simulink model "papersimulation"  (R2023b)
settings: Solver=VariableStepAuto  StartTime=0.0  StopTime=50  RelTol=1e-3
InitFcn:
  | clc;clear;close all
  | Aa = [
  |     -0.026373    0.12687    -12.926     -32.169;
  |     -0.25009    -0.80174    220.55      -0.16307;
  |     0.000171    -0.00754    -0.5510     -0.000334;
  |     0           0           1           0
  | ];
  | 
  | ba = [
  |     0.010887;
  |     -0.18577;
  |     -0.022966;
  |     0
  | ];
  | 
  | ca = [
  |     0    0    0    1
  | ];
  | Am=Aa;
  | bm=ba;
  | cm=ca;
  | K1m = [0.003614, -0.306976, 262.056954, 999.941914]';
  | 
  | theta1 = [7.654562; 6.881398; -1.386117];       % 3x1 vector
  | theta2 = [-4434.189351; -5958.822119; -2550.603134]; % 3x1 vector
  | theta20 = 595.409427;                            % Scalar
  | 
  | theta31 = [-7.654459; -6.860858; 1.385877];     % 3x1 vector
  | theta32 = [4434.169641; 5958.808248; 2550.58291]; % 3x1 vector
  | theta33 = -595.40843;                            % Scalar
  | theta34 = 0.998522;
  | theta= [
  |     theta1;
  |     theta2;
  |     theta20;
  |     theta31;
  |     theta32;
  |     theta33;
  |     theta34
  | ];
  | %initial condition
  | theta0=1.1*theta;
  | kp =-0.023;
  | rho0=1.1*kp;
  | %other constant parameters
  | gamma = 5;
  | alpha = 5;
  | Gamma = alpha*eye(length(theta0));
  | sgnkp = -1;
StopFcn:
  | plot(out.tout,out.y,LineWidth=1.5)
  | hold on
  | plot(out.tout,out.ym,LineWidth=1.5)
  | legend(["$y$","$y_m$"],FontSize=18,Interpreter="latex")
  | xlabel("time",FontSize=18,Interpreter="latex")
  | ylim([-0.5 0.5])
  | grid on
  | 
  | figure
  | plot(out.tout,out.u,LineWidth=1.5)
  | legend("Control signal",FontSize=18,Interpreter="latex")
  | xlabel("time",FontSize=18,Interpreter="latex")
  | grid on
  | 
  | figure
  | plot(out.tout,out.e,LineWidth=1.5)
  | legend("Error",FontSize=18,Interpreter="latex")
  | xlabel("time",FontSize=18,Interpreter="latex")
  | ylim([-0.2 0.6])
  | grid on
settings Model: Creator=IHC  LastModifiedBy=IHC

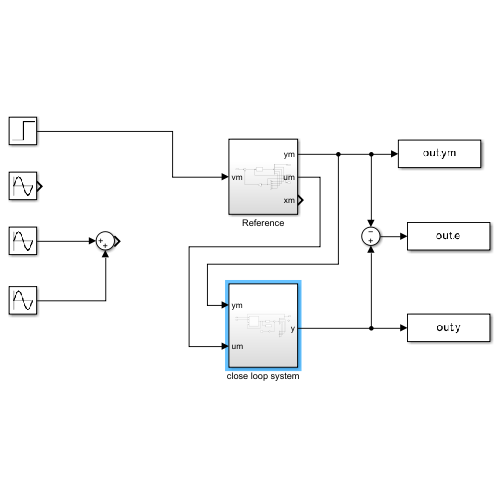
[thumbnail: Simulink's stored preview of the top-level diagram]
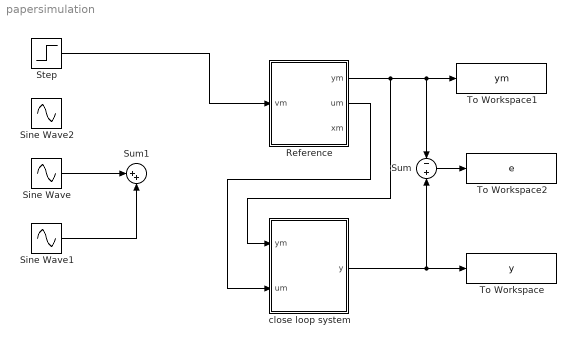
== system papersimulation ==
  Reference : Subsystem
  Sine Wave : Sin  Amplitude=300  Frequency=0.3  SampleTime=0
  Sine Wave1 : Sin  Amplitude=250  Frequency=0.5  SampleTime=0
  Sine Wave2 : Sin  Amplitude=300  Frequency=0.3  SampleTime=0
  Step : Step  Time=0  After=300  SampleTime=0
  Sum : Sum  Inputs=-+
  Sum1 : Sum  Inputs=|++
  To Workspace : ToWorkspace  VariableName=y  SampleTime=-1
  To Workspace1 : ToWorkspace  VariableName=ym  SampleTime=-1
  To Workspace2 : ToWorkspace  VariableName=e  SampleTime=-1
  close loop system : Subsystem
  wires:
  close loop system/1(y) -> To Workspace/1, Sum/2
  Reference/2(um) -> close loop system/2(um)
  Reference/1(ym) -> Sum/1, To Workspace1/1, close loop system/1(ym)
  Sum/1 -> To Workspace2/1
  Sine Wave1/1 -> Sum1/2
  Sine Wave/1 -> Sum1/1
  Step/1 -> Reference/1(vm)

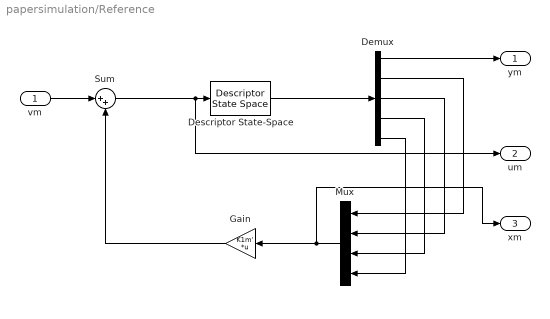
== system papersimulation/Reference ==
  vm : Inport
  Demux : Demux  Outputs=5
  Descriptor State-Space : DescriptorStateSpace  E=eye(4,4)  A=Am  B=bm  C=[cm;eye(4,4)];  D=[0; zeros(4,1)]  InitialCondition=[0;0;0;0]
  Gain : Gain  Gain=K1m'  Multiplication=Matrix(K*u)
  Mux : Mux
  Sum : Sum  Inputs=|++
  ym : Outport
  um : Outport  Port=2
  xm : Outport  Port=3
  wires:
  Descriptor State-Space/1 -> Demux/1
  Demux/2 -> Mux/1
  Demux/3 -> Mux/2
  Demux/4 -> Mux/3
  Demux/5 -> Mux/4
  Demux/1 -> ym/1
  Mux/1 -> Gain/1, xm/1
  vm/1 -> Sum/1
  Sum/1 -> um/1, Descriptor State-Space/1
  Gain/1 -> Sum/2

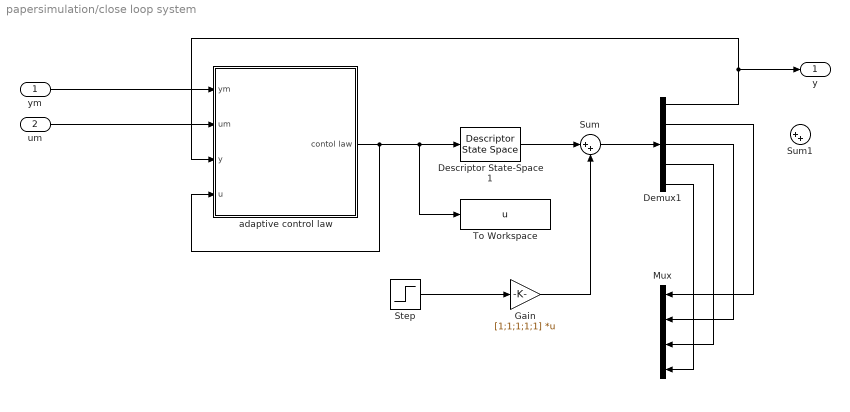
== system papersimulation/close loop system ==
  ym : Inport
  um : Inport  Port=2
  Demux1 : Demux  Outputs=5
  Descriptor State-Space1 : DescriptorStateSpace  E=eye(4,4)  A=Aa  B=ba  C=[ca;eye(4,4)];  D=[0; zeros(4,1)]  InitialCondition=[0;0;0;0.5]
  Gain : Gain  Gain=[1;1;1;1;1]  Multiplication=Matrix(K*u)
  Mux : Mux
  Step : Step  Time=0  After=0.5  SampleTime=0
  Sum : Sum  Inputs=|++
  Sum1 : Sum  Inputs=|++
  To Workspace : ToWorkspace  VariableName=u  SampleTime=-1
  adaptive control law : Subsystem
  y : Outport
  wires:
  Demux1/2 -> Mux/1
  Demux1/3 -> Mux/2
  Demux1/4 -> Mux/3
  Demux1/5 -> Mux/4
  Demux1/1 -> adaptive control law/3(y), y/1
  ym/1 -> adaptive control law/1(ym)
  um/1 -> adaptive control law/2(um)
  adaptive control law/1(contol law) -> To Workspace/1, Descriptor State-Space1/1, adaptive control law/4(u)
  Descriptor State-Space1/1 -> Sum/1
  Sum/1 -> Demux1/1
  Step/1 -> Gain/1
  Gain/1 -> Sum/2

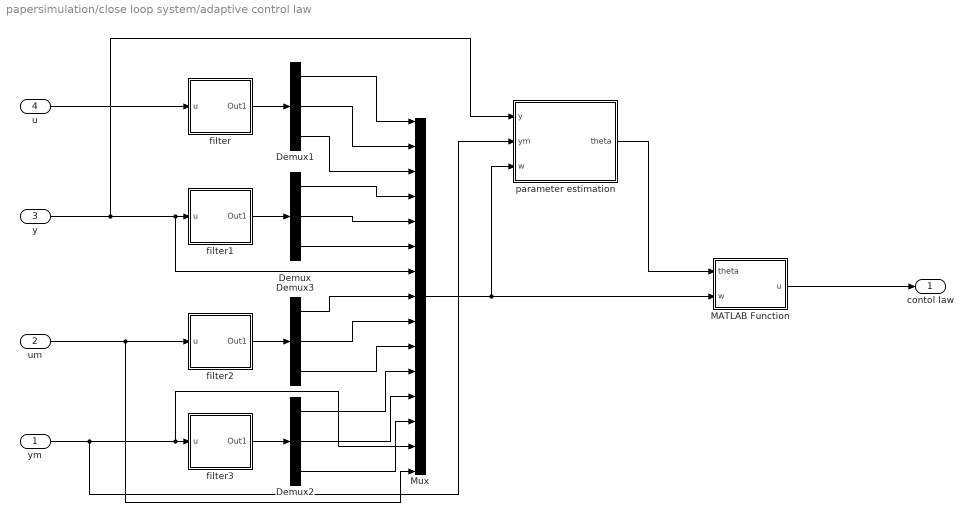
== system papersimulation/close loop system/adaptive control law ==
  ym : Inport
  um : Inport  Port=2
  y : Inport  Port=3
  u : Inport  Port=4
  Demux{,1..3} (4 alike) : Demux  Outputs=3
  MATLAB Function : MATLAB Function  TreatAsAtomicUnit=on
  Mux : Mux  Inputs=15
  filter : Subsystem
  filter1 : Subsystem
  filter2 : Subsystem
  filter3 : Subsystem
  parameter estimation : Subsystem
  contol law : Outport
  wires:
  u/1 -> filter/1(u)
  y/1 -> parameter estimation/1(y), Mux/7, filter1/1(u)
  um/1 -> filter2/1(u), Mux/15
  ym/1 -> parameter estimation/2(ym), Mux/14, filter3/1(u)
  Mux/1 -> MATLAB Function/2(w), parameter estimation/3(w)
  MATLAB Function/1(u) -> contol law/1
  filter3/1(Out1) -> Demux2/1
  filter/1(Out1) -> Demux1/1
  filter1/1(Out1) -> Demux/1
  filter2/1(Out1) -> Demux3/1
  Demux1/1 -> Mux/1
  Demux1/2 -> Mux/2
  Demux1/3 -> Mux/3
  Demux/1 -> Mux/4
  Demux/2 -> Mux/5
  Demux/3 -> Mux/6
  Demux3/1 -> Mux/8
  Demux3/2 -> Mux/9
  Demux3/3 -> Mux/10
  Demux2/1 -> Mux/11
  Demux2/2 -> Mux/12
  Demux2/3 -> Mux/13
  parameter estimation/1(theta) -> MATLAB Function/1(theta)

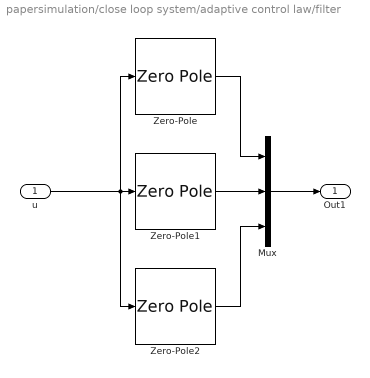
== system papersimulation/close loop system/adaptive control law/filter ==
  u : Inport
  Mux : Mux  Inputs=3
  Zero-Pole : ZeroPole  Zeros=[]  Poles=[-2 -2 -2]
  Zero-Pole1 : ZeroPole  Zeros=[0]  Poles=[-2 -2 -2]
  Zero-Pole2 : ZeroPole  Zeros=[0 0]  Poles=[-2 -2 -2]
  Out1 : Outport
  wires:
  u/1 -> Zero-Pole2/1, Zero-Pole/1, Zero-Pole1/1
  Zero-Pole1/1 -> Mux/2
  Zero-Pole/1 -> Mux/1
  Zero-Pole2/1 -> Mux/3
  Mux/1 -> Out1/1

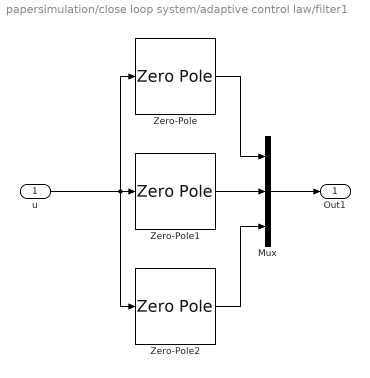
== system papersimulation/close loop system/adaptive control law/filter1 ==
  u : Inport
  Mux : Mux  Inputs=3
  Zero-Pole : ZeroPole  Zeros=[]  Poles=[-2 -2 -2]
  Zero-Pole1 : ZeroPole  Zeros=[0]  Poles=[-2 -2 -2]
  Zero-Pole2 : ZeroPole  Zeros=[0 0]  Poles=[-2 -2 -2]
  Out1 : Outport
  wires:
  u/1 -> Zero-Pole2/1, Zero-Pole/1, Zero-Pole1/1
  Zero-Pole1/1 -> Mux/2
  Zero-Pole/1 -> Mux/1
  Zero-Pole2/1 -> Mux/3
  Mux/1 -> Out1/1

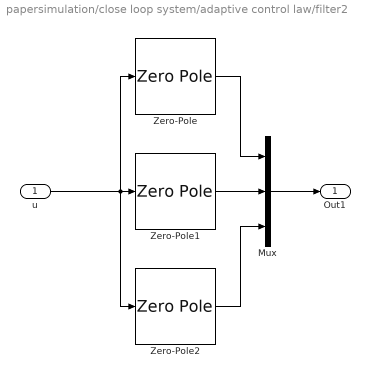
== system papersimulation/close loop system/adaptive control law/filter2 ==
  u : Inport
  Mux : Mux  Inputs=3
  Zero-Pole : ZeroPole  Zeros=[]  Poles=[-2 -2 -2]
  Zero-Pole1 : ZeroPole  Zeros=[0]  Poles=[-2 -2 -2]
  Zero-Pole2 : ZeroPole  Zeros=[0 0]  Poles=[-2 -2 -2]
  Out1 : Outport
  wires:
  u/1 -> Zero-Pole2/1, Zero-Pole/1, Zero-Pole1/1
  Zero-Pole1/1 -> Mux/2
  Zero-Pole/1 -> Mux/1
  Zero-Pole2/1 -> Mux/3
  Mux/1 -> Out1/1

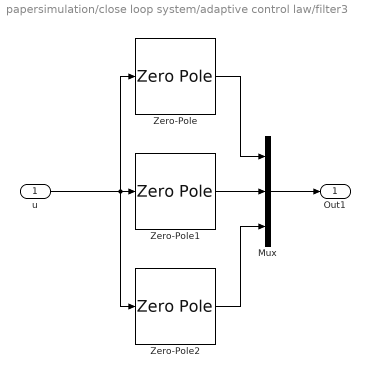
== system papersimulation/close loop system/adaptive control law/filter3 ==
  u : Inport
  Mux : Mux  Inputs=3
  Zero-Pole : ZeroPole  Zeros=[]  Poles=[-2 -2 -2]
  Zero-Pole1 : ZeroPole  Zeros=[0]  Poles=[-2 -2 -2]
  Zero-Pole2 : ZeroPole  Zeros=[0 0]  Poles=[-2 -2 -2]
  Out1 : Outport
  wires:
  u/1 -> Zero-Pole2/1, Zero-Pole/1, Zero-Pole1/1
  Zero-Pole1/1 -> Mux/2
  Zero-Pole/1 -> Mux/1
  Zero-Pole2/1 -> Mux/3
  Mux/1 -> Out1/1

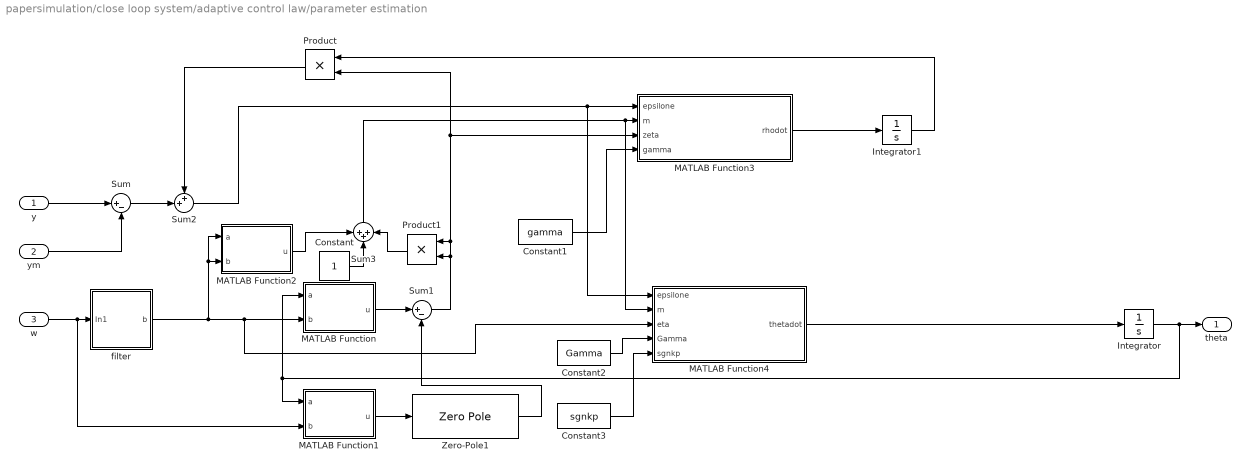
== system papersimulation/close loop system/adaptive control law/parameter estimation ==
  y : Inport
  ym : Inport  Port=2
  w : Inport  Port=3
  Constant : Constant
  Constant1 : Constant  Value=gamma
  Constant2 : Constant  Value=Gamma
  Constant3 : Constant  Value=sgnkp
  Integrator : Integrator  InitialCondition=theta0
  Integrator1 : Integrator  InitialCondition=rho0
  MATLAB Function : MATLAB Function  TreatAsAtomicUnit=on
  MATLAB Function1 : MATLAB Function  TreatAsAtomicUnit=on
  MATLAB Function2 : MATLAB Function  TreatAsAtomicUnit=on
  MATLAB Function3 : MATLAB Function  TreatAsAtomicUnit=on
  MATLAB Function4 : MATLAB Function  TreatAsAtomicUnit=on
  Product : Product
  Product1 : Product
  Sum : Sum  Inputs=|+-
  Sum1 : Sum  Inputs=|+-
  Sum2 : Sum  Inputs=++|
  Sum3 : Sum  Inputs=+++
  Zero-Pole1 : ZeroPole  Zeros=[]  Poles=[-1 -1]
  filter : Subsystem
  theta : Outport
  wires:
  y/1 -> Sum/1
  ym/1 -> Sum/2
  Integrator/1 -> MATLAB Function1/1(a), MATLAB Function/1(a), theta/1
  w/1 -> filter/1(In1), MATLAB Function1/2(b)
  filter/1(b) -> MATLAB Function2/1(a), MATLAB Function2/2(b), MATLAB Function4/3(eta), MATLAB Function/2(b)
  MATLAB Function1/1(u) -> Zero-Pole1/1
  MATLAB Function/1(u) -> Sum1/1
  Zero-Pole1/1 -> Sum1/2
  Integrator1/1 -> Product/1
  Sum1/1 -> MATLAB Function3/3(zeta), Product/2, Product1/1, Product1/2
  Product/1 -> Sum2/1
  Sum/1 -> Sum2/2
  Product1/1 -> Sum3/3
  MATLAB Function2/1(u) -> Sum3/1
  Constant/1 -> Sum3/2
  Sum2/1 -> MATLAB Function4/1(epsilone), MATLAB Function3/1(epsilone)
  Sum3/1 -> MATLAB Function4/2(m), MATLAB Function3/2(m)
  MATLAB Function3/1(rhodot) -> Integrator1/1
  MATLAB Function4/1(thetadot) -> Integrator/1
  Constant1/1 -> MATLAB Function3/4(gamma)
  Constant2/1 -> MATLAB Function4/4(Gamma)
  Constant3/1 -> MATLAB Function4/5(sgnkp)

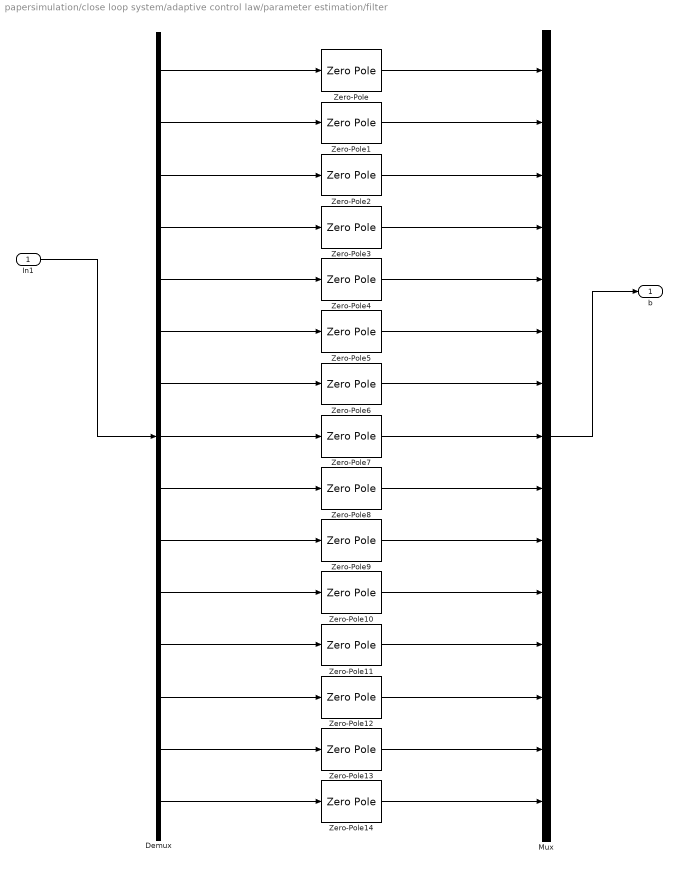
== system papersimulation/close loop system/adaptive control law/parameter estimation/filter ==
  In1 : Inport
  Demux : Demux  Outputs=15
  Mux : Mux  Inputs=15
  Zero-Pole{,1..14} (15 alike) : ZeroPole  Zeros=[]  Poles=[-1 -1]
  b : Outport
  wires:
  Mux/1 -> b/1
  Demux/1 -> Zero-Pole/1
  Demux/2 -> Zero-Pole1/1
  Demux/3 -> Zero-Pole2/1
  Demux/4 -> Zero-Pole3/1
  Demux/5 -> Zero-Pole4/1
  Demux/6 -> Zero-Pole5/1
  Demux/7 -> Zero-Pole6/1
  Demux/8 -> Zero-Pole7/1
  Demux/9 -> Zero-Pole8/1
  Demux/10 -> Zero-Pole9/1
  Demux/11 -> Zero-Pole10/1
  Demux/12 -> Zero-Pole11/1
  Demux/13 -> Zero-Pole12/1
  Demux/14 -> Zero-Pole13/1
  Demux/15 -> Zero-Pole14/1
  Zero-Pole14/1 -> Mux/15
  Zero-Pole13/1 -> Mux/14
  Zero-Pole12/1 -> Mux/13
  Zero-Pole11/1 -> Mux/12
  Zero-Pole10/1 -> Mux/11
  Zero-Pole9/1 -> Mux/10
  Zero-Pole8/1 -> Mux/9
  Zero-Pole7/1 -> Mux/8
  Zero-Pole6/1 -> Mux/7
  Zero-Pole/1 -> Mux/1
  Zero-Pole1/1 -> Mux/2
  Zero-Pole2/1 -> Mux/3
  Zero-Pole3/1 -> Mux/4
  Zero-Pole4/1 -> Mux/5
  Zero-Pole5/1 -> Mux/6
  In1/1 -> Demux/1

== matlab function papersimulation/close loop system/adaptive control law/parameter estimation/MATLAB Function ==
  data: a input; u output; b input
function u = dot(a,b)

u = a'*b;

== matlab function papersimulation/close loop system/adaptive control law/MATLAB Function ==
  data: theta input; u output; w input
function u = dot(theta,w)

u = theta'*w;

== matlab function papersimulation/close loop system/adaptive control law/parameter estimation/MATLAB Function1 ==
  data: a input; u output; b input
function u = dot(a,b)

u = a'*b;;

== matlab function papersimulation/close loop system/adaptive control law/parameter estimation/MATLAB Function2 ==
  data: a input; u output; b input
function u = dot(a,b)

u = a'*b;;

== matlab function papersimulation/close loop system/adaptive control law/parameter estimation/MATLAB Function3 ==
  data: epsilone input; m input; rhodot output; zeta input; gamma input
function rhodot = rho(epsilone,m,zeta,gamma)
rhodot = -gamma*zeta*epsilone/m;

== matlab function papersimulation/close loop system/adaptive control law/parameter estimation/MATLAB Function4 ==
  data: epsilone input; m input; eta input; thetadot output; Gamma input; sgnkp input
function thetadot = Theta(epsilone,m,eta,Gamma,sgnkp)
thetadot = -sgnkp*(Gamma*epsilone/m)*eta;
